simulink model "que2"  (R2016a)
settings: Solver=VariableStepAuto  StartTime=0.0  StopTime=10.0  RelTol=1e-3
undefined symbols (not defined in the file): A, B, C, K2, x0
settings Model: Creator=X1  LastModifiedBy=X1

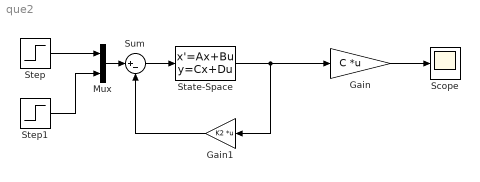
== system que2 ==
  Gain : Gain  Gain=C  Multiplication=Matrix(K*u)
  Gain1 : Gain  Gain=K2  Multiplication=Matrix(K*u)
  Mux : Mux  Inputs=2
  Scope : Scope
  State-Space : StateSpace  A=A  B=B  C=eye(6)  D=zeros(6,2)  X0=x0
  Step : Step  SampleTime=0
  Step1 : Step  SampleTime=0
  Sum : Sum  Inputs=|+-
  wires:
  State-Space/1 -> Gain1/1, Gain/1
  Step/1 -> Mux/1
  Step1/1 -> Mux/2
  Sum/1 -> State-Space/1
  Gain1/1 -> Sum/2
  Gain/1 -> Scope/1
  Mux/1 -> Sum/1
